simulink model "formation"  (R2018b)
settings: Solver=VariableStepAuto  StartTime=0.0  StopTime=10.0  RelTol=1e-3
values from neighbouring files (symbols this model uses):
  dist_des = ones(n, n)-eye(n)    [Init.m]
  num_neighbors = 2    [Init.m]
undefined symbols (not defined in the file or in its folder): A, q0
settings Model: Creator=miche  LastModifiedBy=miche

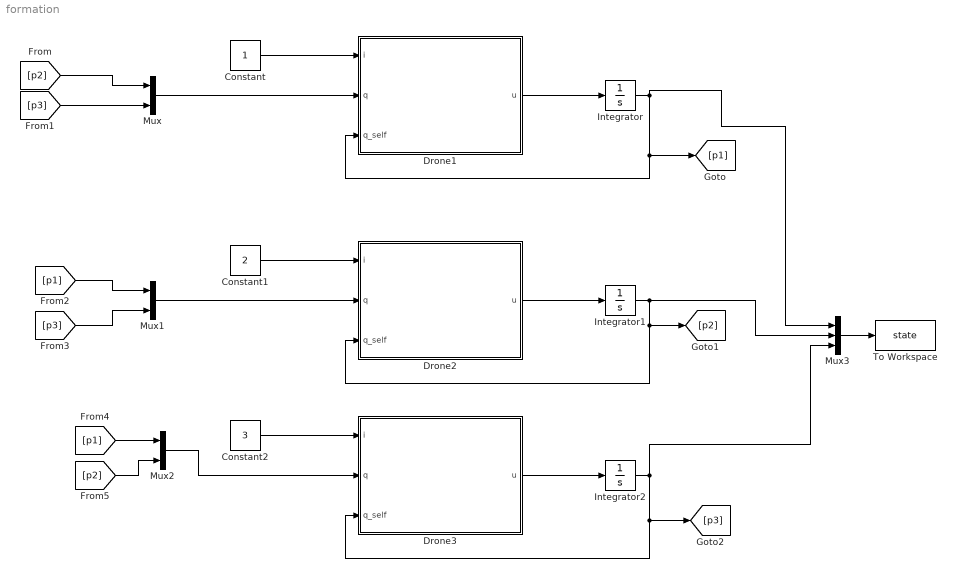
== system formation ==
  Constant : Constant
  Constant1 : Constant  Value=2
  Constant2 : Constant  Value=3
  Drone1 : MATLAB Function  TreatAsAtomicUnit=on
  Drone2 : MATLAB Function  TreatAsAtomicUnit=on
  Drone3 : MATLAB Function  TreatAsAtomicUnit=on
  Integrator : Integrator  InitialCondition=q0(1:3)
  Integrator1 : Integrator  InitialCondition=q0(4:6)
  Integrator2 : Integrator  InitialCondition=q0(7:9)
  Mux : Mux  Inputs=2
  Mux1 : Mux  Inputs=2
  Mux2 : Mux  Inputs=2
  Mux3 : Mux  Inputs=3
  To Workspace : ToWorkspace  VariableName=state  SaveFormat=Timeseries  SampleTime=-1
  wires:
  Drone1/1(u) -> Integrator/1
  Integrator/1 -> [p1], Drone1/3(q_self), Mux3/1
  Constant/1 -> Drone1/1(i)
  Integrator1/1 -> Mux3/2, [p2], Drone2/3(q_self)
  Drone2/1(u) -> Integrator1/1
  Constant1/1 -> Drone2/1(i)
  Integrator2/1 -> [p3], Drone3/3(q_self), Mux3/3
  Drone3/1(u) -> Integrator2/1
  Constant2/1 -> Drone3/1(i)
  Mux/1 -> Drone1/2(q)
  Mux1/1 -> Drone2/2(q)
  [p2] -> Mux/1
  [p3] -> Mux/2
  [p1] -> Mux1/1
  [p3] -> Mux1/2
  [p1] -> Mux2/1
  [p2] -> Mux2/2
  Mux2/1 -> Drone3/2(q)
  Mux3/1 -> To Workspace/1

== matlab function formation/Drone2 ==
  data: u output; A parameter; i input; q input; q_self input; dist_des parameter; num_neighbors parameter
function u = fcn(A, i, q, q_self, dist_des, num_neighbors)
u=[0;0;0];
k=2.5;
    for j=1:1:num_neighbors
        dist=norm(q(j:j+2)-q_self);
        u=u+A(i:i+2,j:j+2)*(q(j:j+2)-q_self)+k*atan(dist-dist_des(i,j:j+2))*(q(j:j+2)-q_self);
    end
end

== matlab function formation/Drone1 ==
  data: u output; A parameter; i input; q input; q_self input; dist_des parameter; num_neighbors parameter
function u = fcn(A, i, q, q_self, dist_des, num_neighbors)
u=[0;0;0];
k=2.5;
    for j=1:1:num_neighbors
        dist=norm(q(j:j+2)-q_self);
        u=u+A(i:i+2,j:j+2)*(q(j:j+2)-q_self)+k*atan(dist-dist_des(i,j:j+2))*(q(j:j+2)-q_self);
    end
end

== matlab function formation/Drone3 ==
  data: u output; A parameter; i input; q input; q_self input; dist_des parameter; num_neighbors parameter
function u = fcn(A, i, q, q_self, dist_des, num_neighbors)
u=[0;0;0];
k=2.5;
    for j=1:1:num_neighbors
        dist=norm(q(j:j+2)-q_self);
        u=u+A(i:i+2,j:j+2)*(q(j:j+2)-q_self)+k*atan(dist-dist_des(i,j:j+2))*(q(j:j+2)-q_self);
    end
end
